simulink model "Ros_PubSub"  (R2020a)
settings: Solver=VariableStepAuto  StartTime=0.0  StopTime=inf  RelTol=1e-3
undefined symbols (not defined in the file or in its folder): Angular, Linear, Pose
libraries: robotlib x9, simulink x4
settings Model: Creator=tatsuyann  LastModifiedBy=tatsuyann

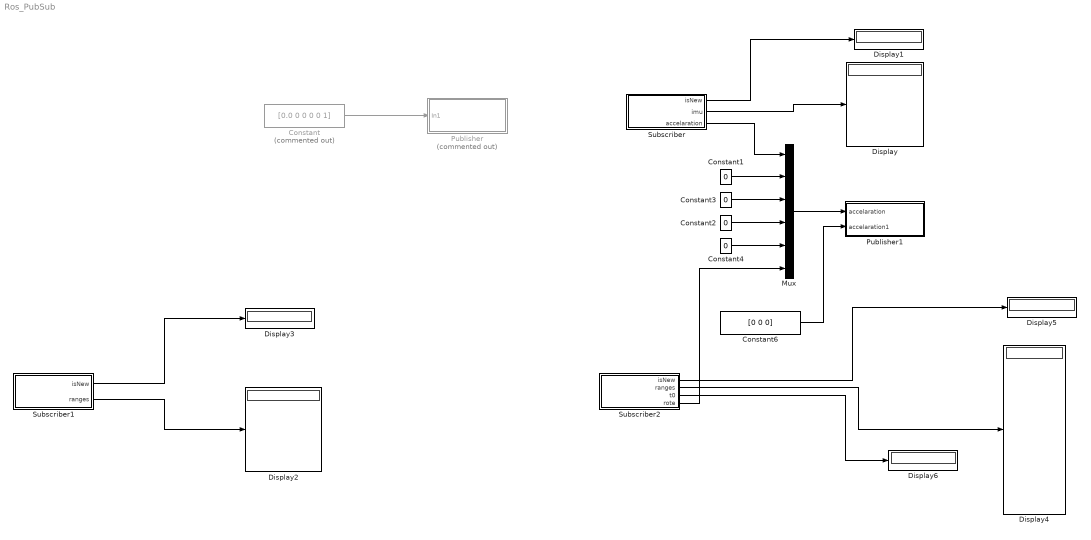
== system Ros_PubSub ==
  Constant : Constant  Commented=on  Value=[0.0 0 0 0 0 1]
  Constant{1..4} (4 alike) : Constant  Value=0
  Constant6 : Constant  Value=[0 0 0]
  Display{,1..6} (7 alike) : Display
  Mux : Mux  Inputs=6
  Publisher : Subsystem  Commented=on
  Publisher1 : Subsystem
  Subscriber : Subsystem
  Subscriber1 : Subsystem
  Subscriber2 : Subsystem
  wires:
  Constant/1 -> Publisher/1(In1)
  Subscriber/2(imu) -> Display/1
  Subscriber/1(isNew) -> Display1/1
  Subscriber1/1(isNew) -> Display3/1
  Subscriber1/2(ranges) -> Display2/1
  Subscriber2/2(ranges) -> Display4/1
  Subscriber2/1(isNew) -> Display5/1
  Mux/1 -> Publisher1/1(accelaration)
  Constant3/1 -> Mux/3
  Subscriber2/4(rote) -> Mux/6
  Constant4/1 -> Mux/5
  Constant2/1 -> Mux/4
  Constant1/1 -> Mux/2
  Subscriber/3(accelaration) -> Mux/1
  Constant6/1 -> Publisher1/2(accelaration1)
  Subscriber2/3(t0) -> Display6/1

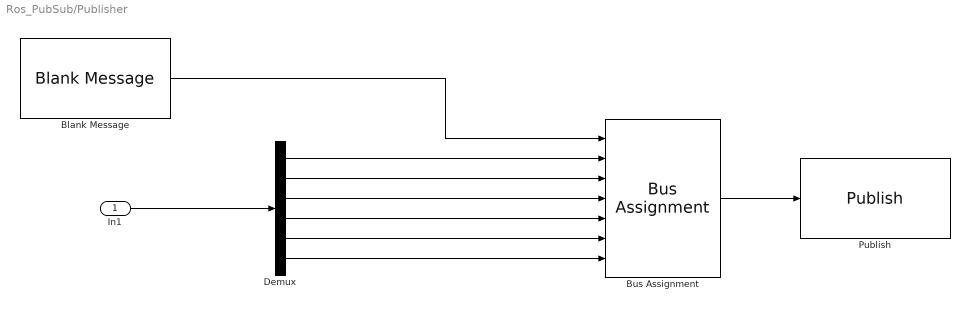
== system Ros_PubSub/Publisher ==
  In1 : Inport
  Blank Message : robotlib/Blank Message  messageClass=Message  entityType=geometry_msgs/Twist  messageType=geometry_msgs/Twist  SampleTime=inf
  Bus Assignment : BusAssignment  AssignedSignals=Linear.X,Linear.Y,Linear.Z,Angular.X,Angular.Y,Angular.Z
  Demux : Demux  Outputs=6
  Publish : robotlib/Publish  topicSource=Specify your own  topic=/cmd_vel  messageType=geometry_msgs/Twist  messageQueueLength=1
  wires:
  In1/1 -> Demux/1
  Blank Message/1 -> Bus Assignment/1
  Demux/6 -> Bus Assignment/7
  Demux/5 -> Bus Assignment/6
  Demux/4 -> Bus Assignment/5
  Demux/3 -> Bus Assignment/4
  Demux/2 -> Bus Assignment/3
  Demux/1 -> Bus Assignment/2
  Bus Assignment/1 -> Publish/1

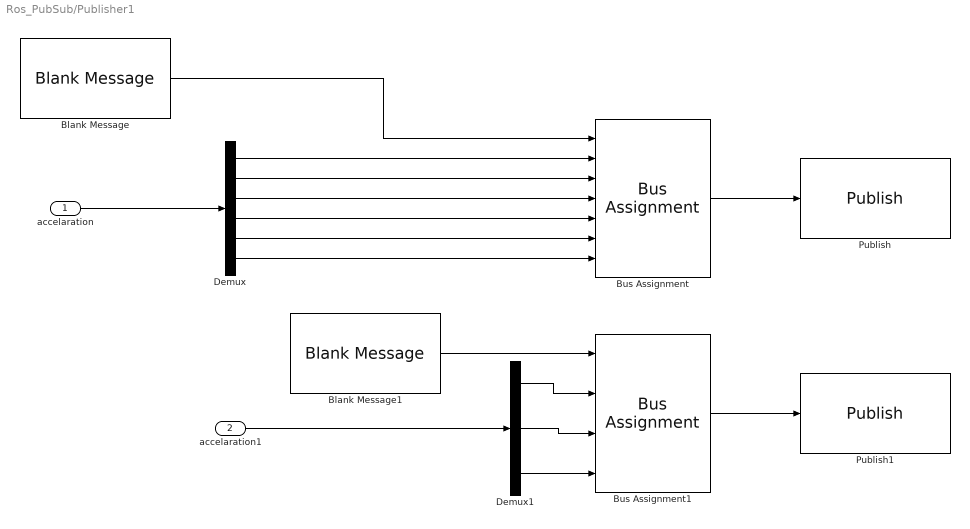
== system Ros_PubSub/Publisher1 ==
  accelaration : Inport
  accelaration1 : Inport  Port=2
  Blank Message : robotlib/Blank Message  messageClass=Message  entityType=geometry_msgs/Twist  messageType=geometry_msgs/Twist  SampleTime=inf
  Blank Message1 : robotlib/Blank Message  messageClass=Message  entityType=nav_msgs/Odometry  messageType=nav_msgs/Odometry  SampleTime=inf
  Bus Assignment : BusAssignment  AssignedSignals=Linear.X,Linear.Y,Linear.Z,Angular.X,Angular.Y,Angular.Z
  Bus Assignment1 : BusAssignment  AssignedSignals=Pose.Pose.Position.X,Pose.Pose.Position.Y,Pose.Pose.Position.Z
  Demux : Demux  Outputs=6
  Demux1 : Demux  Outputs=3
  Publish : robotlib/Publish  topicSource=Specify your own  topic=/cmd_vel  messageType=geometry_msgs/Twist  messageQueueLength=1
  Publish1 : robotlib/Publish  topicSource=Specify your own  topic=/odom  messageType=nav_msgs/Odometry  messageQueueLength=1
  wires:
  Blank Message/1 -> Bus Assignment/1
  Bus Assignment/1 -> Publish/1
  Demux/6 -> Bus Assignment/7
  Demux/1 -> Bus Assignment/2
  Demux/3 -> Bus Assignment/4
  Demux/2 -> Bus Assignment/3
  Demux/4 -> Bus Assignment/5
  accelaration/1 -> Demux/1
  Demux/5 -> Bus Assignment/6
  Blank Message1/1 -> Bus Assignment1/1
  accelaration1/1 -> Demux1/1
  Demux1/1 -> Bus Assignment1/2
  Demux1/2 -> Bus Assignment1/3
  Demux1/3 -> Bus Assignment1/4
  Bus Assignment1/1 -> Publish1/1

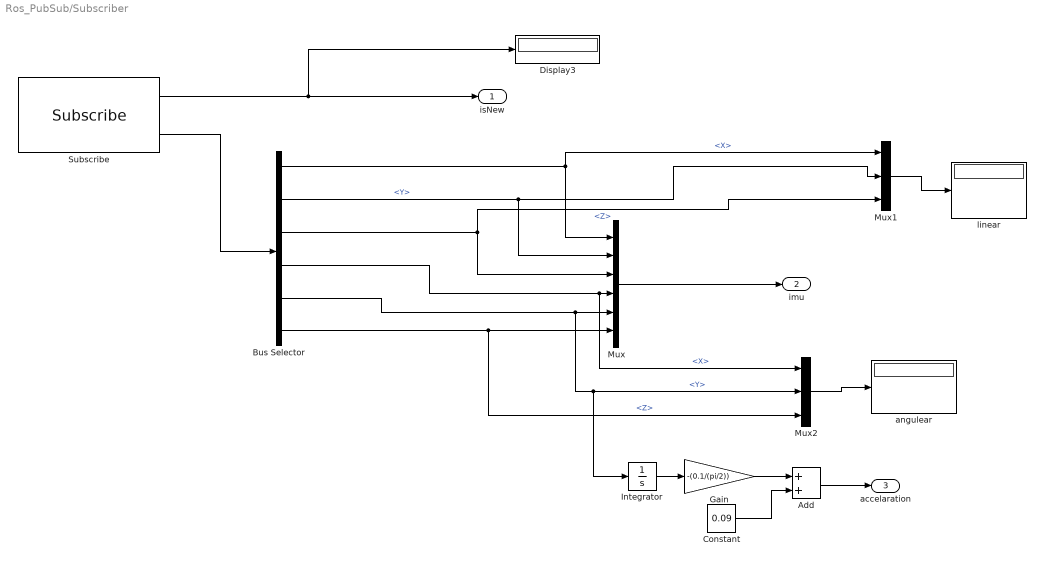
== system Ros_PubSub/Subscriber ==
  Add : Sum
  Bus Selector : BusSelector  OutputSignals=LinearAcceleration.X,LinearAcceleration.Y,LinearAcceleration.Z,AngularVelocity.X,AngularVelocity.Y,AngularVelocity.Z
  Constant : Constant  Value=0.09
  Display3 : Display
  Gain : Gain  Gain=-(0.1/(pi/2))
  Integrator : Integrator
  Mux : Mux  Inputs=6
  Mux1 : Mux  Inputs=3
  Mux2 : Mux  Inputs=3
  Subscribe : robotlib/Subscribe  topicSource=Specify your own  topic=/imu  messageType=sensor_msgs/Imu  sampleTime=0.1  messageQueueLength=1
  angulear : Display
  linear : Display
  isNew : Outport
  imu : Outport  Port=2
  accelaration : Outport  Port=3
  wires:
  Subscribe/2 -> Bus Selector/1
  Bus Selector/3 -> Mux1/3, Mux/3  "<Z>"
  Bus Selector/2 -> Mux1/2, Mux/2  "<Y>"
  Bus Selector/1 -> Mux1/1, Mux/1  "<X>"
  Mux/1 -> imu/1
  Subscribe/1 -> Display3/1, isNew/1
  Bus Selector/4 -> Mux2/1, Mux/4  "<X>"
  Bus Selector/5 -> Integrator/1, Mux2/2, Mux/5  "<Y>"
  Bus Selector/6 -> Mux2/3, Mux/6  "<Z>"
  Mux1/1 -> linear/1
  Mux2/1 -> angulear/1
  Gain/1 -> Add/1
  Constant/1 -> Add/2
  Add/1 -> accelaration/1
  Integrator/1 -> Gain/1

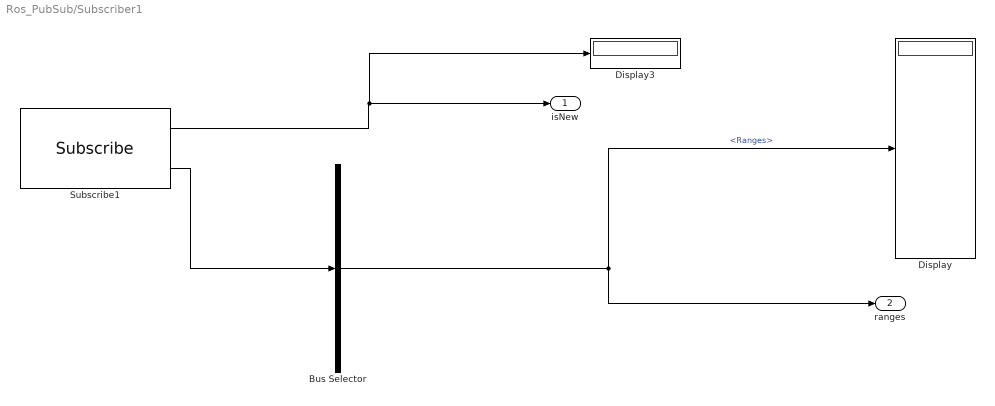
== system Ros_PubSub/Subscriber1 ==
  Bus Selector : BusSelector  OutputSignals=Ranges
  Display : Display
  Display3 : Display
  Subscribe1 : robotlib/Subscribe  topicSource=Specify your own  topic=/scan  messageType=sensor_msgs/LaserScan  sampleTime=0.1  messageQueueLength=1
  isNew : Outport
  ranges : Outport  Port=2
  wires:
  Subscribe1/1 -> Display3/1, isNew/1
  Subscribe1/2 -> Bus Selector/1
  Bus Selector/1 -> Display/1, ranges/1  "<Ranges>"

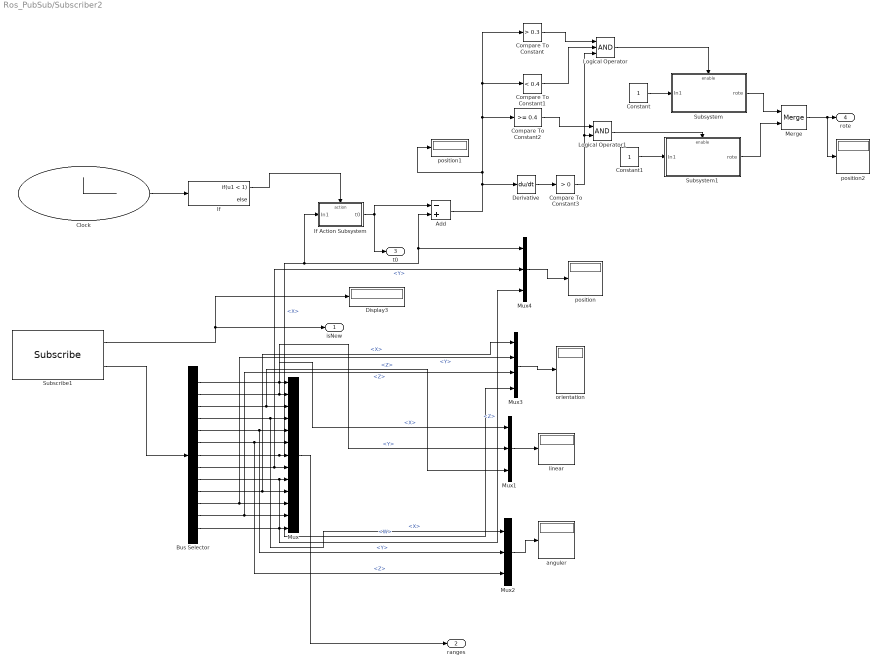
== system Ros_PubSub/Subscriber2 ==
  Add : Sum  Inputs=-+
  Bus Selector : BusSelector  OutputSignals=Twist.Twist.Linear.X,Twist.Twist.Linear.Y,Twist.Twist.Linear.Z,Twist.Twist.Angular.X,Twist.Twist.Angular.Y,Twist.Twist.Angular.Z,Pose.Pose.Position.X,Pose.Pose.Position.Y,Pose.Pose.Position.Z,Pose.Pose.Orientation.X,Pose.Pose.Orientation.Y,Pose.Pose.Orientation.Z,Pose.Pose.Orientation.W
  Clock : Clock
  Compare To Constant : simulink/Logic and Bit Operations/Compare To Constant  relop=>  const=0.3  OutDataTypeStr=boolean
  Compare To Constant1 : simulink/Logic and Bit Operations/Compare To Constant  relop=<  const=0.4  OutDataTypeStr=boolean
  Compare To Constant2 : simulink/Logic and Bit Operations/Compare To Constant  relop=>=  const=0.4  OutDataTypeStr=boolean
  Compare To Constant3 : simulink/Logic and Bit Operations/Compare To Constant  relop=>  const=0  OutDataTypeStr=boolean
  Constant : Constant
  Constant1 : Constant
  Derivative : Derivative
  Display3 : Display
  If : If  IfExpression=u1 < 1
  If Action Subsystem : Subsystem  TreatAsAtomicUnit=on
  Logical Operator : Logic  Inputs=3  AllPortsSameDT=off  OutDataTypeStr=boolean
  Logical Operator1 : Logic  AllPortsSameDT=off  OutDataTypeStr=boolean
  Merge : Merge
  Mux : Mux  Inputs=13
  Mux1 : Mux  Inputs=3
  Mux2 : Mux  Inputs=3
  Mux3 : Mux
  Mux4 : Mux  Inputs=3
  Subscribe1 : robotlib/Subscribe  topicSource=Specify your own  topic=/odom  messageType=nav_msgs/Odometry  sampleTime=0.1  messageQueueLength=1
  Subsystem : Subsystem
  Subsystem1 : Subsystem
  anguler : Display
  linear : Display
  orientation : Display
  position : Display
  position1 : Display
  position2 : Display
  isNew : Outport
  ranges : Outport  Port=2
  t0 : Outport  Port=3
  rote : Outport  Port=4
  wires:
  Subscribe1/1 -> Display3/1, isNew/1
  Subscribe1/2 -> Bus Selector/1
  Mux2/1 -> anguler/1
  Mux1/1 -> linear/1
  Bus Selector/1 -> Mux1/1, Mux/1  "<X>"
  Bus Selector/2 -> Mux1/2, Mux/2  "<Y>"
  Bus Selector/4 -> Mux2/1, Mux/4  "<X>"
  Bus Selector/3 -> Mux1/3, Mux/3  "<Z>"
  Bus Selector/5 -> Mux2/2, Mux/5  "<Y>"
  Bus Selector/6 -> Mux2/3, Mux/6  "<Z>"
  Bus Selector/7 -> If Action Subsystem/1(In1), Mux4/1, Add/2, Mux/7  "<X>"
  Bus Selector/8 -> Mux/8, Mux4/2  "<Y>"
  Bus Selector/9 -> Mux4/3, Mux/9  "<Z>"
  Bus Selector/10 -> Mux/10, Mux3/1  "<X>"
  Bus Selector/11 -> Mux/11, Mux3/2  "<Y>"
  Bus Selector/12 -> Mux3/3, Mux/12  "<Z>"
  Bus Selector/13 -> Mux3/4, Mux/13  "<W>"
  Mux3/1 -> orientation/1
  Mux4/1 -> position/1
  Mux/1 -> ranges/1
  Clock/1 -> If/1
  If/1 -> If Action Subsystem/Action
  If Action Subsystem/1(t0) -> t0/1, Add/1
  Add/1 -> Derivative/1, Compare To Constant2/1, Compare To Constant/1, Compare To Constant1/1, position1/1
  Compare To Constant/1 -> Logical Operator/1
  Compare To Constant1/1 -> Logical Operator/2
  Logical Operator/1 -> Subsystem/Enable
  Constant/1 -> Subsystem/1(In1)
  Constant1/1 -> Subsystem1/1(In1)
  Subsystem1/1(rote) -> Merge/2
  Merge/1 -> position2/1, rote/1
  Subsystem/1(rote) -> Merge/1
  Derivative/1 -> Compare To Constant3/1
  Compare To Constant2/1 -> Logical Operator1/1
  Compare To Constant3/1 -> Logical Operator/3, Logical Operator1/2
  Logical Operator1/1 -> Subsystem1/Enable

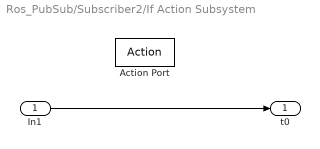
== system Ros_PubSub/Subscriber2/If Action Subsystem ==
  In1 : Inport
  Action Port : ActionPort  ActionPortLabel=if(u1 < 1)
  t0 : Outport
  wires:
  In1/1 -> t0/1

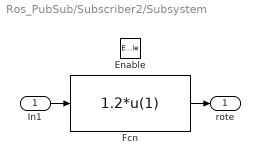
== system Ros_PubSub/Subscriber2/Subsystem ==
  In1 : Inport
  Enable : EnablePort
  Fcn : Fcn  Expr=1.2*u(1)
  rote : Outport
  wires:
  Fcn/1 -> rote/1
  In1/1 -> Fcn/1

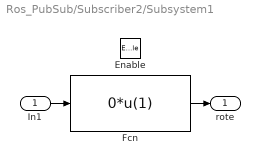
== system Ros_PubSub/Subscriber2/Subsystem1 ==
  In1 : Inport
  Enable : EnablePort
  Fcn : Fcn  Expr=0*u(1)
  rote : Outport
  wires:
  Fcn/1 -> rote/1
  In1/1 -> Fcn/1
